simulink model "PID_Lab2"  (R2023a)
settings: Solver=VariableStepAuto  StartTime=0.0  StopTime=10.0  MaxStep=0.001  RelTol=1e-3
values from neighbouring files (symbols this model uses):
  K = 1.5    [lab2_PID.m]
  T = 0.5    [lab2_PID.m]
  Wn = 8    [lab2_PID.m]
  Zeta = 1    [lab2_PID.m]
settings Model: Creator=alaam  LastModifiedBy=alaam

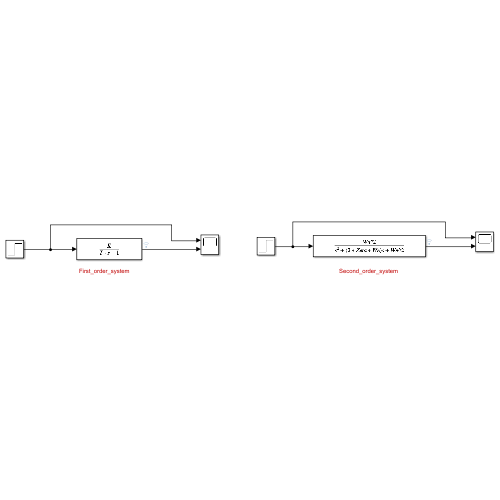
[thumbnail: Simulink's stored preview of the top-level diagram]
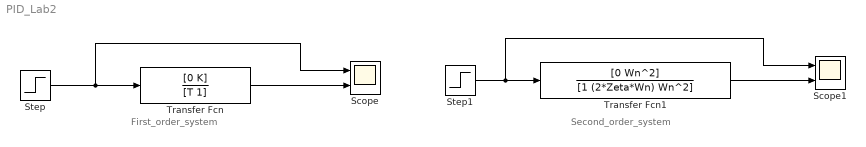
== system PID_Lab2 ==
  note: First_order_system
  note: Second_order_system
  Scope : Scope  NumInputPorts=2
  Scope1 : Scope  NumInputPorts=2
  Step : Step  SampleTime=0
  Step1 : Step  SampleTime=0
  Transfer Fcn : TransferFcn  Numerator=[0 K]  Denominator=[T 1]
  Transfer Fcn1 : TransferFcn  Numerator=[0 Wn^2]  Denominator=[1 (2*Zeta*Wn) Wn^2]
  wires:
  Step/1 -> Scope/1, Transfer Fcn/1
  Transfer Fcn/1 -> Scope/2
  Transfer Fcn1/1 -> Scope1/2
  Step1/1 -> Transfer Fcn1/1, Scope1/1
